simulink model "SYSTEM"  (R2026a)
settings: Solver=VariableStepAuto
model workspace (MAT data in the model file):
  CompAir_P : Simulink.ConnectionBus (value not decoded)
  CompAir_S : Simulink.Bus (value not decoded)
  Control_P : Simulink.ConnectionBus (value not decoded)
  Control_S : Simulink.Bus (value not decoded)
  CoolingFW_P : Simulink.ConnectionBus (value not decoded)
  CoolingFW_S : Simulink.Bus (value not decoded)
  FuelOil_P : Simulink.ConnectionBus (value not decoded)
  FuelOil_S : Simulink.Bus (value not decoded)
  Heat_P : Simulink.ConnectionBus (value not decoded)
  Heat_S : Simulink.Bus (value not decoded)
  LubeOil_P : Simulink.ConnectionBus (value not decoded)
  LubeOil_S : Simulink.Bus (value not decoded)
  Physical : Simulink.ConnectionBus (value not decoded)
  Power_P : Simulink.ConnectionBus (value not decoded)
  Power_S : Simulink.Bus (value not decoded)
  SaltWater_P : Simulink.ConnectionBus (value not decoded)
  SaltWater_S : Simulink.Bus (value not decoded)
  WasteGas_P : Simulink.ConnectionBus (value not decoded)
  WasteGas_S : Simulink.Bus (value not decoded)
  WasteOil_P : Simulink.ConnectionBus (value not decoded)
  WasteOil_S : Simulink.Bus (value not decoded)
  WasteSolid_P : Simulink.ConnectionBus (value not decoded)
  WasteSolid_S : Simulink.Bus (value not decoded)
  WasteWater_P : Simulink.ConnectionBus (value not decoded)
  WasteWater_S : Simulink.Bus (value not decoded)
undefined symbols (not defined in the file): FUEL
(part 2 of 5)

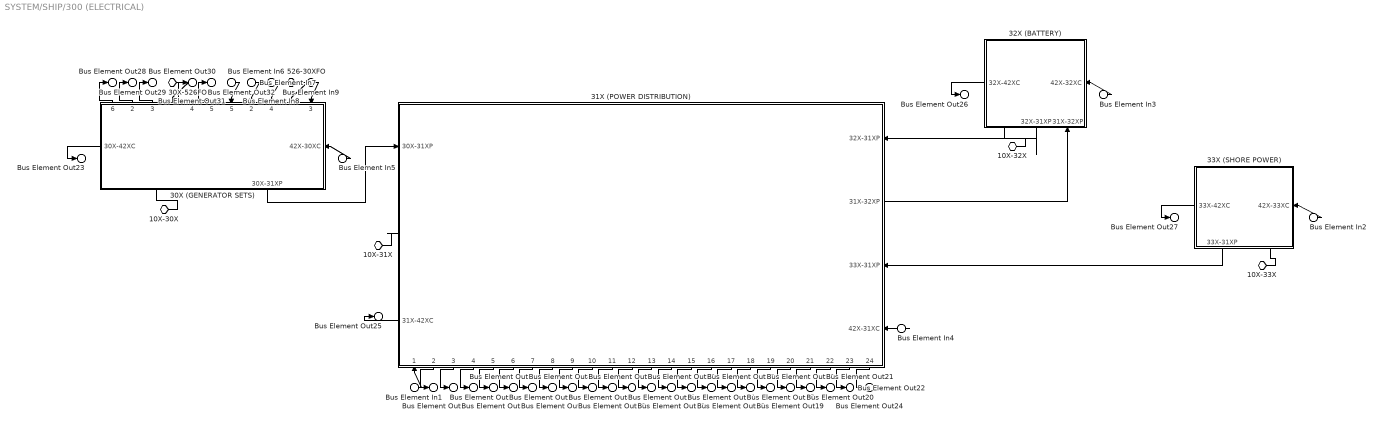
== system SYSTEM/SHIP/300 (ELECTRICAL) ==
  Bus Element In6 : Inport  PortName=50X-30XCFW
  Bus Element In7 : Inport  Port=2  PortName=51X-30XLO
  Bus Element In8 : Inport  Port=3  PortName=52X-30XFO
  Bus Element In9 : Inport  Port=4  PortName=53X-30XCA
  Bus Element In5 : Inport  Port=5  PortName=42X-30XC
  Bus Element In4 : Inport  Port=6  PortName=42X-31XC
  Bus Element In3 : Inport  Port=7  PortName=42X-32XC
  Bus Element In2 : Inport  Port=8  PortName=42X-33XC
  Bus Element In1 : Inport  Port=9  PortName=23X-31XP
  30X (GENERATOR SETS) : Subsystem
      settings: PortSchema="{\"entries\":[{\"content\":{\"headerSize\":26,\"margin\":15,\"minimumSpacing\":25,\"sides\":[{\"content\":{\"connectorIds\":[\"Out1\"]},\"type\":\"ConnectorPlacement.EquallySpacedRectSide\",\"uuid\":\"c62bca68-e99b-4d4a-8c3b-c9a3c6520291\"},{\"content\":{\"connectorIds\":[\"In1\"],\"side\":\"RIGHT\"},\"type\":\"ConnectorPlacement.EquallySpacedRectSide\",\"uuid\":\"9f78cd75-5645-4950-8d66-9f0d33627f1f\"},{\"content\":{\"connectorIds\":[\"Out6\",\"Out2\",\"Out3\",\"LConn1\",\"Out4\",\"Out5\",\"In5\",\"In2\",\"In4\",\"LConn2\",\"In3\"],\"side\":\"TOP\"},\"type\":\"ConnectorPlacement.EquallySpacedRectSide\",\"uuid\":\"f95077c9-4a6b-4bf1-8b13-59697d659817\"},{\"content\":{\"connectorIds\":[\"RConn1\",\"Out7\"],\"side\":\"BOTTOM\"},\"type\":\"ConnectorPlacement.EquallySpacedRectSide\",\"uuid\":\"264ceb2d-2194-473f-bd49-42333d529a66\"}]},\"type\":\"ConnectorPlacement.EquallySpacedConnector\",\"uuid\":\"da1ef182-4ed3-4fb4-823f-e8eb0a5ecd15\"}],\"packageUris\":[\"http://schema.mathworks.com/mf0/Connector/R2020b\"],\"version\":\"1.0\"}"
  31X (POWER DISTRIBUTION) : Subsystem
      settings: PortSchema="{\"entries\":[{\"content\":{\"headerSize\":26,\"margin\":15,\"minimumSpacing\":25,\"sides\":[{\"content\":{\"connectorIds\":[\"In4\",\"RConn1\",\"Out1\"]},\"type\":\"ConnectorPlacement.EquallySpacedRectSide\",\"uuid\":\"c62bca68-e99b-4d4a-8c3b-c9a3c6520291\"},{\"content\":{\"connectorIds\":[\"In2\",\"Out25\",\"In5\",\"In3\"],\"side\":\"RIGHT\"},\"type\":\"ConnectorPlacement.EquallySpacedRectSide\",\"uuid\":\"9f78cd75-5645-4950-8d66-9f0d33627f1f\"},{\"content\":{\"side\":\"TOP\"},\"type\":\"ConnectorPlacement.EquallySpacedRectSide\",\"uuid\":\"f95077c9-4a6b-4bf1-8b13-59697d659817\"},{\"content\":{\"connectorIds\":[\"In1\",\"Out2\",\"Out3\",\"Out4\",\"Out5\",\"Out6\",\"Out7\",\"Out8\",\"Out9\",\"Out10\",\"Out11\",\"Out12\",\"Out13\",\"Out14\",\"Out15\",\"Out16\",\"Out17\",\"Out18\",\"Out19\",\"Out20\",\"Out21\",\"Out22\",\"Out23\",\"Out24\"],\"side\":\"BOTTOM\"},\"type\":\"ConnectorPlacement.EquallySpacedRectSide\",\"uuid\":\"f6dd318a-df87-4470-894a-05aa0d1c9a62\"}]},\"type\":\"ConnectorPlacement.EquallySpacedConnector\",\"uuid\":\"da1ef182-4ed3-4fb4-823f-e8eb0a5ecd15\"}],\"packageUris\":[\"http://schema.mathworks.com/mf0/Connector/R2020b\"],\"version\":\"1.0\"}"
  32X (BATTERY) : Subsystem
      settings: PortSchema="{\"entries\":[{\"content\":{\"headerSize\":26,\"margin\":15,\"minimumSpacing\":25,\"sides\":[{\"content\":{\"connectorIds\":[\"Out2\"]},\"type\":\"ConnectorPlacement.EquallySpacedRectSide\",\"uuid\":\"c62bca68-e99b-4d4a-8c3b-c9a3c6520291\"},{\"content\":{\"connectorIds\":[\"In1\"],\"side\":\"RIGHT\"},\"type\":\"ConnectorPlacement.EquallySpacedRectSide\",\"uuid\":\"9f78cd75-5645-4950-8d66-9f0d33627f1f\"},{\"content\":{\"side\":\"TOP\"},\"type\":\"ConnectorPlacement.EquallySpacedRectSide\",\"uuid\":\"f95077c9-4a6b-4bf1-8b13-59697d659817\"},{\"content\":{\"connectorIds\":[\"RConn1\",\"Out1\",\"In2\"],\"side\":\"BOTTOM\"},\"type\":\"ConnectorPlacement.EquallySpacedRectSide\",\"uuid\":\"3a1d08c9-370f-4ab6-aa25-1f67b2c1fd59\"}]},\"type\":\"ConnectorPlacement.EquallySpacedConnector\",\"uuid\":\"da1ef182-4ed3-4fb4-823f-e8eb0a5ecd15\"}],\"packageUris\":[\"http://schema.mathworks.com/mf0/Connector/R2020b\"],\"version\":\"1.0\"}"
  33X (SHORE POWER) : Subsystem
      settings: PortSchema="{\"entries\":[{\"content\":{\"headerSize\":26,\"margin\":15,\"minimumSpacing\":25,\"sides\":[{\"content\":{\"connectorIds\":[\"Out1\"]},\"type\":\"ConnectorPlacement.EquallySpacedRectSide\",\"uuid\":\"c62bca68-e99b-4d4a-8c3b-c9a3c6520291\"},{\"content\":{\"connectorIds\":[\"In1\"],\"side\":\"RIGHT\"},\"type\":\"ConnectorPlacement.EquallySpacedRectSide\",\"uuid\":\"9f78cd75-5645-4950-8d66-9f0d33627f1f\"},{\"content\":{\"side\":\"TOP\"},\"type\":\"ConnectorPlacement.EquallySpacedRectSide\",\"uuid\":\"f95077c9-4a6b-4bf1-8b13-59697d659817\"},{\"content\":{\"connectorIds\":[\"Out2\",\"RConn1\"],\"side\":\"BOTTOM\"},\"type\":\"ConnectorPlacement.EquallySpacedRectSide\",\"uuid\":\"7c8141e3-2141-4bb3-89bd-e025a2a4dcbf\"}]},\"type\":\"ConnectorPlacement.EquallySpacedConnector\",\"uuid\":\"da1ef182-4ed3-4fb4-823f-e8eb0a5ecd15\"}],\"packageUris\":[\"http://schema.mathworks.com/mf0/Connector/R2020b\"],\"version\":\"1.0\"}"
  30X-526FO : PMIOPort  Side=Left  ConnectionType=Bus: FuelOil_P
  526-30XFO : PMIOPort  Port=2  Side=Left  ConnectionType=Bus: FuelOil_P
  10X-30X : PMIOPort  Port=3  Side=Left  ConnectionType=Bus: Physical
  10X-31X : PMIOPort  Port=4  Side=Left  ConnectionType=Bus: Physical
  10X-32X : PMIOPort  Port=5  Side=Left  ConnectionType=Bus: Physical
  10X-33X : PMIOPort  Port=6  Side=Left  ConnectionType=Bus: Physical
  Bus Element Out28 : Outport  PortName=30X-50XCFW
  Bus Element Out29 : Outport  Port=2  PortName=30X-51XLO
  Bus Element Out30 : Outport  Port=3  PortName=30X-52XFO
  Bus Element Out31 : Outport  Port=4  PortName=30X-53XCA
  Bus Element Out32 : Outport  Port=5  PortName=30X-57XWG
  Bus Element Out23 : Outport  Port=6  PortName=30X-42XC
  Bus Element Out25 : Outport  Port=7  PortName=31X-42XC
  Bus Element Out26 : Outport  Port=8  PortName=32X-42XC
  Bus Element Out27 : Outport  Port=9  PortName=33X-42XC
  Bus Element Out2 : Outport  Port=10  PortName=31X-40XP
  Bus Element Out7 : Outport  Port=11  PortName=31X-41XP
  Bus Element Out3 : Outport  Port=12  PortName=31X-42XP
  Bus Element Out5 : Outport  Port=13  PortName=31X-43XP
  Bus Element Out6 : Outport  Port=14  PortName=31X-44XP
  Bus Element Out4 : Outport  Port=15  PortName=31X-45XP
  Bus Element Out1 : Outport  Port=16  PortName=31X-50XP
  Bus Element Out8 : Outport  Port=17  PortName=31X-51XP
  Bus Element Out9 : Outport  Port=18  PortName=31X-529P
  Bus Element Out10 : Outport  Port=19  PortName=31X-53XP
  Bus Element Out11 : Outport  Port=20  PortName=31X-54XP
  Bus Element Out12 : Outport  Port=21  PortName=31X-55XP
  Bus Element Out13 : Outport  Port=22  PortName=31X-56XP
  Bus Element Out14 : Outport  Port=23  PortName=31X-57XP
  Bus Element Out15 : Outport  Port=24  PortName=31X-58XP
  Bus Element Out16 : Outport  Port=25  PortName=31X-59XP
  Bus Element Out17 : Outport  Port=26  PortName=31X-60XP
  Bus Element Out18 : Outport  Port=27  PortName=31X-61XP
  Bus Element Out19 : Outport  Port=28  PortName=31X-70XP
  Bus Element Out20 : Outport  Port=29  PortName=31X-71XP
  Bus Element Out21 : Outport  Port=30  PortName=31X-72XP
  Bus Element Out22 : Outport  Port=31  PortName=31X-73XP
  Bus Element Out24 : Outport  Port=32  PortName=31X-74XP
  wires:
  30X (GENERATOR SETS)/7(30X-31XP) -> 31X (POWER DISTRIBUTION)/4(30X-31XP)
  33X (SHORE POWER)/2(33X-31XP) -> 31X (POWER DISTRIBUTION)/5(33X-31XP)
  31X (POWER DISTRIBUTION)/25(31X-32XP) -> 32X (BATTERY)/2(31X-32XP)
  32X (BATTERY)/1(32X-31XP) -> 31X (POWER DISTRIBUTION)/2(32X-31XP)
  Bus Element In1/1 -> 31X (POWER DISTRIBUTION)/1(23X-31XP)
  31X (POWER DISTRIBUTION)/2(31X-40XP) -> Bus Element Out2/1
  31X (POWER DISTRIBUTION)/3(31X-41XP) -> Bus Element Out7/1
  31X (POWER DISTRIBUTION)/4(31X-42XP) -> Bus Element Out3/1
  31X (POWER DISTRIBUTION)/5(31X-43XP) -> Bus Element Out5/1
  31X (POWER DISTRIBUTION)/6(31X-44XP) -> Bus Element Out6/1
  31X (POWER DISTRIBUTION)/7(31X-45XP) -> Bus Element Out4/1
  31X (POWER DISTRIBUTION)/8(31X-50XP) -> Bus Element Out1/1
  31X (POWER DISTRIBUTION)/9(31X-51XP) -> Bus Element Out8/1
  31X (POWER DISTRIBUTION)/10(31X-529P) -> Bus Element Out9/1
  31X (POWER DISTRIBUTION)/11(31X-53XP) -> Bus Element Out10/1
  31X (POWER DISTRIBUTION)/12(31X-54XP) -> Bus Element Out11/1
  31X (POWER DISTRIBUTION)/13(31X-55XP) -> Bus Element Out12/1
  31X (POWER DISTRIBUTION)/14(31X-56XP) -> Bus Element Out13/1
  31X (POWER DISTRIBUTION)/15(31X-57XP) -> Bus Element Out14/1
  31X (POWER DISTRIBUTION)/16(31X-58XP) -> Bus Element Out15/1
  31X (POWER DISTRIBUTION)/17(31X-59XP) -> Bus Element Out16/1
  31X (POWER DISTRIBUTION)/18(31X-60XP) -> Bus Element Out17/1
  31X (POWER DISTRIBUTION)/19(31X-61XP) -> Bus Element Out18/1
  31X (POWER DISTRIBUTION)/20(31X-70XP) -> Bus Element Out19/1
  31X (POWER DISTRIBUTION)/21(31X-71XP) -> Bus Element Out20/1
  31X (POWER DISTRIBUTION)/22(31X-72XP) -> Bus Element Out21/1
  31X (POWER DISTRIBUTION)/23(31X-73XP) -> Bus Element Out22/1
  31X (POWER DISTRIBUTION)/24(31X-74XP) -> Bus Element Out24/1
  Bus Element In5/1 -> 30X (GENERATOR SETS)/1(42X-30XC)
  Bus Element In4/1 -> 31X (POWER DISTRIBUTION)/3(42X-31XC)
  Bus Element In3/1 -> 32X (BATTERY)/1(42X-32XC)
  Bus Element In2/1 -> 33X (SHORE POWER)/1(42X-33XC)
  30X (GENERATOR SETS)/1(30X-42XC) -> Bus Element Out23/1
  31X (POWER DISTRIBUTION)/1(31X-42XC) -> Bus Element Out25/1
  32X (BATTERY)/2(32X-42XC) -> Bus Element Out26/1
  33X (SHORE POWER)/1(33X-42XC) -> Bus Element Out27/1
  30X (GENERATOR SETS)/6(30X-50XCFW) -> Bus Element Out28/1
  Bus Element In6/1 -> 30X (GENERATOR SETS)/5(50X-30XCFW)
  30X (GENERATOR SETS)/2(30X-51XLO) -> Bus Element Out29/1
  Bus Element In7/1 -> 30X (GENERATOR SETS)/2(51X-30XLO)
  30X (GENERATOR SETS)/3(30X-52XFO) -> Bus Element Out30/1
  Bus Element In8/1 -> 30X (GENERATOR SETS)/4(52X-30XFO)
  30X (GENERATOR SETS)/4(30X-53XCA) -> Bus Element Out31/1
  Bus Element In9/1 -> 30X (GENERATOR SETS)/3(53X-30XCA)
  30X (GENERATOR SETS)/5(30X-57XWG) -> Bus Element Out32/1
  connections:
  30X (GENERATOR SETS)/RConn1 -- 10X-30X/RConn1
  31X (POWER DISTRIBUTION)/RConn1 -- 10X-31X/RConn1
  32X (BATTERY)/RConn1 -- 10X-32X/RConn1
  33X (SHORE POWER)/RConn1 -- 10X-33X/RConn1
  30X-526FO/RConn1 -- 30X (GENERATOR SETS)/LConn1
  526-30XFO/RConn1 -- 30X (GENERATOR SETS)/LConn2

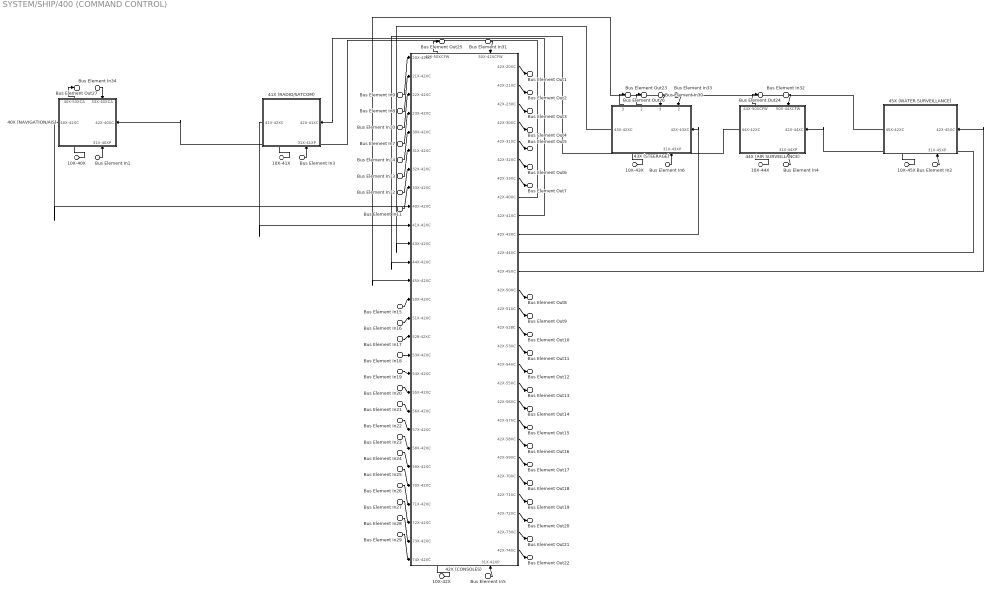
== system SYSTEM/SHIP/400 (COMMAND CONTROL) ==
  Bus Element In31 : Inport  PortName=50X-42XCFW
  Bus Element In32 : Inport  Port=2  PortName=50X-44XCFW
  Bus Element In30 : Inport  Port=3  PortName=50X-43XCFW
  Bus Element In33 : Inport  Port=4  PortName=51X-43XLO
  Bus Element In34 : Inport  Port=5  PortName=53X-40XCA
  Bus Element In14 : Inport  Port=6  PortName=30X-42XC
  Bus Element In13 : Inport  Port=7  PortName=31X-42XC
  Bus Element In12 : Inport  Port=8  PortName=32X-42XC
  Bus Element In11 : Inport  Port=9  PortName=33X-42XC
  Bus Element In9 : Inport  Port=10  PortName=20X-42XC
  Bus Element In8 : Inport  Port=11  PortName=21X-42XC
  Bus Element In10 : Inport  Port=12  PortName=22X-42XC
  Bus Element In7 : Inport  Port=13  PortName=23X-42XC
  Bus Element In15 : Inport  Port=14  PortName=50X-42XC
  Bus Element In16 : Inport  Port=15  PortName=51X-42XC
  Bus Element In17 : Inport  Port=16  PortName=528-42XC
  Bus Element In18 : Inport  Port=17  PortName=53X-42XC
  Bus Element In19 : Inport  Port=18  PortName=54X-42XC
  Bus Element In20 : Inport  Port=19  PortName=55X-42XC
  Bus Element In21 : Inport  Port=20  PortName=56X-42XC
  Bus Element In22 : Inport  Port=21  PortName=57X-42XC
  Bus Element In23 : Inport  Port=22  PortName=58X-42XC
  Bus Element In24 : Inport  Port=23  PortName=59X-42XC
  Bus Element In25 : Inport  Port=24  PortName=70X-42XC
  Bus Element In26 : Inport  Port=25  PortName=71X-42XC
  Bus Element In27 : Inport  Port=26  PortName=72X-42XC
  Bus Element In28 : Inport  Port=27  PortName=73X-42XC
  Bus Element In29 : Inport  Port=28  PortName=74X-42XC
  Bus Element In1 : Inport  Port=29  PortName=31X-40XP
  Bus Element In3 : Inport  Port=30  PortName=31X-41XP
  Bus Element In5 : Inport  Port=31  PortName=31X-42XP
  Bus Element In6 : Inport  Port=32  PortName=31X-43XP
  Bus Element In4 : Inport  Port=33  PortName=31X-44XP
  Bus Element In2 : Inport  Port=34  PortName=31X-45XP
  40X (NAVIGATION/AIS) : Subsystem
      settings: PortSchema="{\"entries\":[{\"content\":{\"headerSize\":26,\"margin\":15,\"minimumSpacing\":25,\"sides\":[{\"content\":{\"connectorIds\":[\"Out2\"]},\"type\":\"ConnectorPlacement.EquallySpacedRectSide\",\"uuid\":\"c62bca68-e99b-4d4a-8c3b-c9a3c6520291\"},{\"content\":{\"connectorIds\":[\"In2\"],\"side\":\"RIGHT\"},\"type\":\"ConnectorPlacement.EquallySpacedRectSide\",\"uuid\":\"9f78cd75-5645-4950-8d66-9f0d33627f1f\"},{\"content\":{\"connectorIds\":[\"Out1\",\"In1\"],\"side\":\"TOP\"},\"type\":\"ConnectorPlacement.EquallySpacedRectSide\",\"uuid\":\"f95077c9-4a6b-4bf1-8b13-59697d659817\"},{\"content\":{\"connectorIds\":[\"RConn1\",\"In3\"],\"side\":\"BOTTOM\"},\"type\":\"ConnectorPlacement.EquallySpacedRectSide\",\"uuid\":\"81423529-a1bc-46e6-bc40-f3387860b642\"}]},\"type\":\"ConnectorPlacement.EquallySpacedConnector\",\"uuid\":\"da1ef182-4ed3-4fb4-823f-e8eb0a5ecd15\"}],\"packageUris\":[\"http://schema.mathworks.com/mf0/Connector/R2020b\"],\"version\":\"1.0\"}"
  41X (RADIO/SATCOM) : Subsystem
      settings: PortSchema="{\"entries\":[{\"content\":{\"headerSize\":26,\"margin\":15,\"minimumSpacing\":25,\"sides\":[{\"content\":{\"connectorIds\":[\"Out1\"]},\"type\":\"ConnectorPlacement.EquallySpacedRectSide\",\"uuid\":\"c62bca68-e99b-4d4a-8c3b-c9a3c6520291\"},{\"content\":{\"connectorIds\":[\"In1\"],\"side\":\"RIGHT\"},\"type\":\"ConnectorPlacement.EquallySpacedRectSide\",\"uuid\":\"9f78cd75-5645-4950-8d66-9f0d33627f1f\"},{\"content\":{\"side\":\"TOP\"},\"type\":\"ConnectorPlacement.EquallySpacedRectSide\",\"uuid\":\"f95077c9-4a6b-4bf1-8b13-59697d659817\"},{\"content\":{\"connectorIds\":[\"RConn1\",\"In2\"],\"side\":\"BOTTOM\"},\"type\":\"ConnectorPlacement.EquallySpacedRectSide\",\"uuid\":\"da139d07-68bb-432f-9238-27bb23eab08f\"}]},\"type\":\"ConnectorPlacement.EquallySpacedConnector\",\"uuid\":\"da1ef182-4ed3-4fb4-823f-e8eb0a5ecd15\"}],\"packageUris\":[\"http://schema.mathworks.com/mf0/Connector/R2020b\"],\"version\":\"1.0\"}"
  42X (CONSOLES) : Subsystem
      settings: PortSchema="{\"entries\":[{\"content\":{\"headerSize\":26,\"margin\":15,\"minimumSpacing\":25,\"sides\":[{\"content\":{\"connectorIds\":[\"In7\",\"In8\",\"In9\",\"In10\",\"In11\",\"In12\",\"In13\",\"In14\",\"In3\",\"In2\",\"In4\",\"In5\",\"In6\",\"In15\",\"In16\",\"In17\",\"In18\",\"In19\",\"In20\",\"In21\",\"In22\",\"In23\",\"In24\",\"In25\",\"In26\",\"In27\",\"In28\",\"In29\"]},\"type\":\"ConnectorPlacement.EquallySpacedRectSide\",\"uuid\":\"c62bca68-e99b-4d4a-8c3b-c9a3c6520291\"},{\"content\":{\"connectorIds\":[\"Out7\",\"Out8\",\"Out9\",\"Out10\",\"Out11\",\"Out12\",\"Out13\",\"Out2\",\"Out3\",\"Out4\",\"Out5\",\"Out6\",\"Out14\",\"Out15\",\"Out16\",\"Out17\",\"Out18\",\"Out19\",\"Out20\",\"Out21\",\"Out22\",\"Out23\",\"Out24\",\"Out25\",\"Out26\",\"Out27\",\"Out28\"],\"side\":\"RIGHT\"},\"type\":\"ConnectorPlacement.EquallySpacedRectSide\",\"uuid\":\"9f78cd75-5645-4950-8d66-9f0d33627f1f\"},{\"content\":{\"connectorIds\":[\"Out1\",\"In1\"],\"side\":\"TOP\"},\"type\":\"ConnectorPlacement.EquallySpacedRectSide\",\"uuid\":\"f95077c9-4a6b-4bf1-8b13-59697d659817\"},{\"content\":{\"connectorIds\":[\"RConn1\",\"In30\"],\"side\":\"BOTTOM\"},\"type\":\"ConnectorPlacement.EquallySpacedRectSide\",\"uuid\":\"1fb75e57-0aa7-47b9-9db9-f1720a956b48\"}]},\"type\":\"ConnectorPlacement.EquallySpacedConnector\",\"uuid\":\"da1ef182-4ed3-4fb4-823f-e8eb0a5ecd15\"}],\"packageUris\":[\"http://schema.mathworks.com/mf0/Connector/R2020b\"],\"version\":\"1.0\"}"
  43X (STEERAGE) : Subsystem
      settings: PortSchema="{\"entries\":[{\"content\":{\"headerSize\":26,\"margin\":15,\"minimumSpacing\":25,\"sides\":[{\"content\":{\"connectorIds\":[\"Out1\"]},\"type\":\"ConnectorPlacement.EquallySpacedRectSide\",\"uuid\":\"c62bca68-e99b-4d4a-8c3b-c9a3c6520291\"},{\"content\":{\"connectorIds\":[\"In1\"],\"side\":\"RIGHT\"},\"type\":\"ConnectorPlacement.EquallySpacedRectSide\",\"uuid\":\"9f78cd75-5645-4950-8d66-9f0d33627f1f\"},{\"content\":{\"connectorIds\":[\"Out3\",\"Out2\",\"In3\",\"In2\"],\"side\":\"TOP\"},\"type\":\"ConnectorPlacement.EquallySpacedRectSide\",\"uuid\":\"f95077c9-4a6b-4bf1-8b13-59697d659817\"},{\"content\":{\"connectorIds\":[\"RConn1\",\"In4\"],\"side\":\"BOTTOM\"},\"type\":\"ConnectorPlacement.EquallySpacedRectSide\",\"uuid\":\"d3cc4164-1d39-4472-8fd9-8021e77ef95a\"}]},\"type\":\"ConnectorPlacement.EquallySpacedConnector\",\"uuid\":\"da1ef182-4ed3-4fb4-823f-e8eb0a5ecd15\"}],\"packageUris\":[\"http://schema.mathworks.com/mf0/Connector/R2020b\"],\"version\":\"1.0\"}"
  44X (AIR SURVEILLANCE) : Subsystem
      settings: PortSchema="{\"entries\":[{\"content\":{\"headerSize\":26,\"margin\":15,\"minimumSpacing\":25,\"sides\":[{\"content\":{\"connectorIds\":[\"Out2\"]},\"type\":\"ConnectorPlacement.EquallySpacedRectSide\",\"uuid\":\"c62bca68-e99b-4d4a-8c3b-c9a3c6520291\"},{\"content\":{\"connectorIds\":[\"In2\"],\"side\":\"RIGHT\"},\"type\":\"ConnectorPlacement.EquallySpacedRectSide\",\"uuid\":\"9f78cd75-5645-4950-8d66-9f0d33627f1f\"},{\"content\":{\"connectorIds\":[\"Out1\",\"In1\"],\"side\":\"TOP\"},\"type\":\"ConnectorPlacement.EquallySpacedRectSide\",\"uuid\":\"f95077c9-4a6b-4bf1-8b13-59697d659817\"},{\"content\":{\"connectorIds\":[\"RConn1\",\"In3\"],\"side\":\"BOTTOM\"},\"type\":\"ConnectorPlacement.EquallySpacedRectSide\",\"uuid\":\"41665955-c6de-4230-afea-9a8839b333a2\"}]},\"type\":\"ConnectorPlacement.EquallySpacedConnector\",\"uuid\":\"da1ef182-4ed3-4fb4-823f-e8eb0a5ecd15\"}],\"packageUris\":[\"http://schema.mathworks.com/mf0/Connector/R2020b\"],\"version\":\"1.0\"}"
  45X (WATER SURVEILLANCE) : Subsystem
      settings: PortSchema="{\"entries\":[{\"content\":{\"headerSize\":26,\"margin\":15,\"minimumSpacing\":25,\"sides\":[{\"content\":{\"connectorIds\":[\"Out1\"]},\"type\":\"ConnectorPlacement.EquallySpacedRectSide\",\"uuid\":\"c62bca68-e99b-4d4a-8c3b-c9a3c6520291\"},{\"content\":{\"connectorIds\":[\"In1\"],\"side\":\"RIGHT\"},\"type\":\"ConnectorPlacement.EquallySpacedRectSide\",\"uuid\":\"9f78cd75-5645-4950-8d66-9f0d33627f1f\"},{\"content\":{\"side\":\"TOP\"},\"type\":\"ConnectorPlacement.EquallySpacedRectSide\",\"uuid\":\"f95077c9-4a6b-4bf1-8b13-59697d659817\"},{\"content\":{\"connectorIds\":[\"RConn1\",\"In2\"],\"side\":\"BOTTOM\"},\"type\":\"ConnectorPlacement.EquallySpacedRectSide\",\"uuid\":\"f04420a7-4858-4183-a869-fa956f6b3c21\"}]},\"type\":\"ConnectorPlacement.EquallySpacedConnector\",\"uuid\":\"da1ef182-4ed3-4fb4-823f-e8eb0a5ecd15\"}],\"packageUris\":[\"http://schema.mathworks.com/mf0/Connector/R2020b\"],\"version\":\"1.0\"}"
  10X-40X : PMIOPort  Side=Left  ConnectionType=Bus: Physical
  10X-41X : PMIOPort  Port=2  Side=Left  ConnectionType=Bus: Physical
  10X-42X : PMIOPort  Port=3  Side=Left  ConnectionType=Bus: Physical
  10X-43X : PMIOPort  Port=4  Side=Left  ConnectionType=Bus: Physical
  10X-44X : PMIOPort  Port=5  Side=Left  ConnectionType=Bus: Physical
  10X-45X : PMIOPort  Port=6  Side=Left  ConnectionType=Bus: Physical
  Bus Element Out27 : Outport  PortName=40X-53XCA
  Bus Element Out23 : Outport  Port=2  PortName=43X-50XCFW
  Bus Element Out25 : Outport  Port=3  PortName=42X-50XCFW
  Bus Element Out26 : Outport  Port=4  PortName=43X-51XLO
  Bus Element Out24 : Outport  Port=5  PortName=44X-50XCFW
  Bus Element Out1 : Outport  Port=6  PortName=42X-20XC
  Bus Element Out2 : Outport  Port=7  PortName=42X-21XC
  Bus Element Out3 : Outport  Port=8  PortName=42X-23XC
  Bus Element Out4 : Outport  Port=9  PortName=42X-30XC
  Bus Element Out5 : Outport  Port=10  PortName=42X-31XC
  Bus Element Out6 : Outport  Port=11  PortName=42X-32XC
  Bus Element Out7 : Outport  Port=12  PortName=42X-33XC
  Bus Element Out8 : Outport  Port=13  PortName=42X-50XC
  Bus Element Out9 : Outport  Port=14  PortName=42X-51XC
  Bus Element Out10 : Outport  Port=15  PortName=42X-528C
  Bus Element Out11 : Outport  Port=16  PortName=42X-53XC
  Bus Element Out12 : Outport  Port=17  PortName=42X-54XC
  Bus Element Out13 : Outport  Port=18  PortName=42X-55XC
  Bus Element Out14 : Outport  Port=19  PortName=42X-56XC
  Bus Element Out15 : Outport  Port=20  PortName=42X-57XC
  Bus Element Out16 : Outport  Port=21  PortName=42X-58XC
  Bus Element Out17 : Outport  Port=22  PortName=42X-59XC
  Bus Element Out18 : Outport  Port=23  PortName=42X-70XC
  Bus Element Out19 : Outport  Port=24  PortName=42X-71XC
  Bus Element Out20 : Outport  Port=25  PortName=42X-72XC
  Bus Element Out21 : Outport  Port=26  PortName=42X-73XC
  Bus Element Out22 : Outport  Port=27  PortName=42X-74XC
  wires:
  Bus Element In1/1 -> 40X (NAVIGATION/AIS)/3(31X-40XP)
  Bus Element In3/1 -> 41X (RADIO/SATCOM)/2(31X-41XP)
  Bus Element In5/1 -> 42X (CONSOLES)/30(31X-42XP)
  Bus Element In6/1 -> 43X (STEERAGE)/4(31X-43XP)
  Bus Element In4/1 -> 44X (AIR SURVEILLANCE)/3(31X-44XP)
  Bus Element In2/1 -> 45X (WATER SURVEILLANCE)/2(31X-45XP)
  40X (NAVIGATION/AIS)/2(40X-42XC) -> 42X (CONSOLES)/3(40X-42XC)
  41X (RADIO/SATCOM)/1(41X-42XC) -> 42X (CONSOLES)/2(41X-42XC)
  43X (STEERAGE)/1(43X-42XC) -> 42X (CONSOLES)/4(43X-42XC)
  44X (AIR SURVEILLANCE)/2(44X-42XC) -> 42X (CONSOLES)/5(44X-42XC)
  45X (WATER SURVEILLANCE)/1(45X-42XC) -> 42X (CONSOLES)/6(45X-42XC)
  42X (CONSOLES)/2(42X-40XC) -> 40X (NAVIGATION/AIS)/2(42X-40XC)
  42X (CONSOLES)/3(42X-41XC) -> 41X (RADIO/SATCOM)/1(42X-41XC)
  42X (CONSOLES)/4(42X-43XC) -> 43X (STEERAGE)/1(42X-43XC)
  42X (CONSOLES)/5(42X-44XC) -> 44X (AIR SURVEILLANCE)/2(42X-44XC)
  42X (CONSOLES)/6(42X-45XC) -> 45X (WATER SURVEILLANCE)/1(42X-45XC)
  Bus Element In9/1 -> 42X (CONSOLES)/7(20X-42XC)
  Bus Element In8/1 -> 42X (CONSOLES)/8(21X-42XC)
  Bus Element In7/1 -> 42X (CONSOLES)/10(23X-42XC)
  42X (CONSOLES)/7(42X-20XC) -> Bus Element Out1/1
  42X (CONSOLES)/8(42X-21XC) -> Bus Element Out2/1
  42X (CONSOLES)/9(42X-23XC) -> Bus Element Out3/1
  Bus Element In10/1 -> 42X (CONSOLES)/9(22X-42XC)
  42X (CONSOLES)/10(42X-30XC) -> Bus Element Out4/1
  42X (CONSOLES)/11(42X-31XC) -> Bus Element Out5/1
  42X (CONSOLES)/12(42X-32XC) -> Bus Element Out6/1
  42X (CONSOLES)/13(42X-33XC) -> Bus Element Out7/1
  Bus Element In14/1 -> 42X (CONSOLES)/11(30X-42XC)
  Bus Element In13/1 -> 42X (CONSOLES)/12(31X-42XC)
  Bus Element In12/1 -> 42X (CONSOLES)/13(32X-42XC)
  Bus Element In11/1 -> 42X (CONSOLES)/14(33X-42XC)
  42X (CONSOLES)/14(42X-50XC) -> Bus Element Out8/1
  42X (CONSOLES)/15(42X-51XC) -> Bus Element Out9/1
  42X (CONSOLES)/16(42X-528C) -> Bus Element Out10/1
  42X (CONSOLES)/17(42X-53XC) -> Bus Element Out11/1
  42X (CONSOLES)/18(42X-54XC) -> Bus Element Out12/1
  42X (CONSOLES)/19(42X-55XC) -> Bus Element Out13/1
  42X (CONSOLES)/20(42X-56XC) -> Bus Element Out14/1
  42X (CONSOLES)/21(42X-57XC) -> Bus Element Out15/1
  42X (CONSOLES)/22(42X-58XC) -> Bus Element Out16/1
  42X (CONSOLES)/23(42X-59XC) -> Bus Element Out17/1
  Bus Element In15/1 -> 42X (CONSOLES)/15(50X-42XC)
  Bus Element In16/1 -> 42X (CONSOLES)/16(51X-42XC)
  Bus Element In17/1 -> 42X (CONSOLES)/17(528-42XC)
  Bus Element In18/1 -> 42X (CONSOLES)/18(53X-42XC)
  Bus Element In19/1 -> 42X (CONSOLES)/19(54X-42XC)
  Bus Element In20/1 -> 42X (CONSOLES)/20(55X-42XC)
  Bus Element In21/1 -> 42X (CONSOLES)/21(56X-42XC)
  Bus Element In22/1 -> 42X (CONSOLES)/22(57X-42XC)
  Bus Element In23/1 -> 42X (CONSOLES)/23(58X-42XC)
  Bus Element In24/1 -> 42X (CONSOLES)/24(59X-42XC)
  Bus Element In25/1 -> 42X (CONSOLES)/25(70X-42XC)
  Bus Element In26/1 -> 42X (CONSOLES)/26(71X-42XC)
  Bus Element In27/1 -> 42X (CONSOLES)/27(72X-42XC)
  Bus Element In28/1 -> 42X (CONSOLES)/28(73X-42XC)
  Bus Element In29/1 -> 42X (CONSOLES)/29(74X-42XC)
  42X (CONSOLES)/24(42X-70XC) -> Bus Element Out18/1
  42X (CONSOLES)/25(42X-71XC) -> Bus Element Out19/1
  42X (CONSOLES)/26(42X-72XC) -> Bus Element Out20/1
  42X (CONSOLES)/27(42X-73XC) -> Bus Element Out21/1
  42X (CONSOLES)/28(42X-74XC) -> Bus Element Out22/1
  43X (STEERAGE)/3(43X-50XCFW) -> Bus Element Out23/1
  Bus Element In30/1 -> 43X (STEERAGE)/3(50X-43XCFW)
  42X (CONSOLES)/1(42X-50XCFW) -> Bus Element Out25/1
  44X (AIR SURVEILLANCE)/1(44X-50XCFW) -> Bus Element Out24/1
  Bus Element In31/1 -> 42X (CONSOLES)/1(50X-42XCFW)
  Bus Element In32/1 -> 44X (AIR SURVEILLANCE)/1(50X-44XCFW)
  43X (STEERAGE)/2(43X-51XLO) -> Bus Element Out26/1
  Bus Element In33/1 -> 43X (STEERAGE)/2(51X-43XLO)
  Bus Element In34/1 -> 40X (NAVIGATION/AIS)/1(53X-40XCA)
  40X (NAVIGATION/AIS)/1(40X-53XCA) -> Bus Element Out27/1
  connections:
  40X (NAVIGATION/AIS)/RConn1 -- 10X-40X/RConn1
  41X (RADIO/SATCOM)/RConn1 -- 10X-41X/RConn1
  42X (CONSOLES)/RConn1 -- 10X-42X/RConn1
  43X (STEERAGE)/RConn1 -- 10X-43X/RConn1
  44X (AIR SURVEILLANCE)/RConn1 -- 10X-44X/RConn1
  45X (WATER SURVEILLANCE)/RConn1 -- 10X-45X/RConn1
